simulink model "BFBAdsorber"  (Simulink 7.8)
settings: Solver=FixedStepDiscrete  StartTime=0.0  StopTime=100  FixedStep=10  RelTol=1e-5  AbsTol=1e-5
values from neighbouring files (symbols this model uses):
  up = u_plant    [SimulatePlant.m]
settings Model: Creator=pmahapatra  LastModifiedBy=pmahapatra
settings OptimizationCC: BlockReduction=off  BooleanDataType=off  InlineInvariantSignals=on  InitFltsAndDblsToZero=on
settings DebuggingCC: SaveWithParameterizedLinksMsg=none  SignalResolutionControl=TryResolveAllWithWarning  SolverPrmCheckMsg=none  MultiTaskDSMMsg=warning  MultiTaskCondExecSysMsg=none  FcnCallInpInsideContextMsg=Use local settings  StrictBusMsg=None
settings RTWCC: IncludeERTFirstTime=on
settings GRTTargetCC: TargetFcnLib=ansi_tfl_tmw.mat

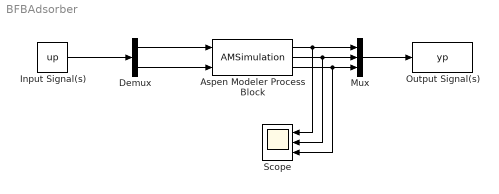
== system BFBAdsorber ==
  Aspen Modeler Process Block : M-S-Function  LoadFcn=|  FunctionName=AMSimulation  Parameters='C:\Program Files\CCSI\APC Framework\Examples\BFB_Adsorber\BFBAdsorberDyn_v5.1.1.acmf','ACM Application',2,'B2.Input_\B1.Input_',3,'CO2_Capture_Percent.Output_\VALVE3.SorbIn.Fm|kg/hr\VALVE1.GasIn.F|kmol/hr',true,false,false
      | LoadModel=actxserver('AMSimulation.Control');
      | invoke(LoadModel,'LoadModel',get_param(gcb,'Parameters'),pwd);
      | LoadModel.delete;
      settings: DeleteFcn=|
      | CloseModel=actxserver('AMSimulation.Control');
      | invoke(CloseModel,'CloseModel',get_param(gcb,'Parameters'));
      | CloseModel.delete;
      settings: OpenFcn=|
      | SetupGUI=actxserver('AMSimulation.Setup');
      | NewParam=invoke(SetupGUI,'SetupModel',get_param(gcb,'Parameters'),pwd,get_param(gcb,'Name'));
      | set_param(gcb,'Parameters',NewParam);
      | SetupGUI.delete;
  Demux : Demux  Outputs=2
  Input Signal(s) : Constant  Value=up
  Mux : Mux  Inputs=3
  Output Signal(s) : ToWorkspace  VariableName=yp  SampleTime=-1  SaveFormat=Array
  Scope : Scope  NumInputPorts=3
      settings: YMin=-5~-5~-5  YMax=5~5~5
  wires:
  Demux/1 -> Aspen Modeler Process Block/1
  Demux/2 -> Aspen Modeler Process Block/2
  Input Signal(s)/1 -> Demux/1
  Aspen Modeler Process Block/1 -> Mux/1, Scope/1
  Aspen Modeler Process Block/2 -> Mux/2, Scope/2
  Mux/1 -> Output Signal(s)/1
  Aspen Modeler Process Block/3 -> Mux/3, Scope/3
